simulink model "lmi_robust_maglev"  (R2018a)
settings: Solver=VariableStepAuto  StartTime=0.0  StopTime=5  RelTol=1e-3
settings Model: Creator=saad  LastModifiedBy=saad

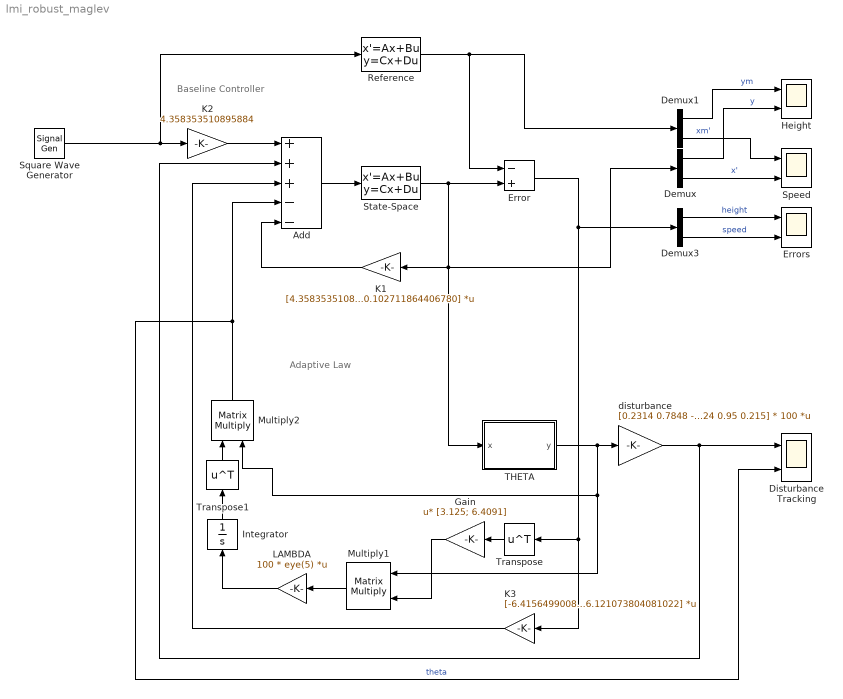
== system lmi_robust_maglev ==
  note: Adaptive Law
  note: Baseline Controller
  Add : Sum  Inputs=+++--
  Demux : Demux  Outputs=2
  Demux1 : Demux  Outputs=2
  Demux3 : Demux  Outputs=2
  Disturbance Tracking : Scope  NumInputPorts=2
  Error : Sum  Inputs=-+
  Errors : Scope  NumInputPorts=2
  Gain : Gain  Gain=[3.125; 6.4091]  Multiplication=Matrix(u*K)
  Height : Scope  NumInputPorts=2
  Integrator : Integrator
  K1 : Gain  Gain=[4.358353510895883,0.102711864406780]  Multiplication=Matrix(K*u)
  K2 : Gain  Gain=4.358353510895884
  K3 : Gain  Gain=[-6.415649900832197,-6.121073804081022]  Multiplication=Matrix(K*u)
  LAMBDA : Gain  Gain=100 * eye(5)  Multiplication=Matrix(K*u)
  Multiply1 : Product  Multiplication=Matrix(*)
  Multiply2 : Product  Multiplication=Matrix(*)
  Reference : StateSpace  A=[0,1;-3600,-84.839999999999990]  B=[0;3600]  C=eye(2)  D=[0;0]  InitialCondition=0  ContinuousStateAttributes={'angle', 'angular_speed'}
  Speed : Scope  NumInputPorts=2
  Square Wave Generator : SignalGenerator  WaveForm=square  Amplitude=-1
  State-Space : StateSpace  A=[0 1;0 0]  B=[0;826]  C=eye(2)  D=[0;0]  InitialCondition=0  ContinuousStateAttributes={'angle', 'angular_speed'}
  THETA : MATLAB Function  TreatAsAtomicUnit=on
  Transpose : Math  Operator=transpose  SaturateOnIntegerOverflow=on
  Transpose1 : Math  Operator=transpose  SaturateOnIntegerOverflow=on
  disturbance : Gain  Gain=[0.2314 0.7848 -0.624 0.95 0.215] * 100  Multiplication=Matrix(K*u)
  wires:
  Add/1 -> State-Space/1
  Square Wave Generator/1 -> Reference/1, K2/1
  K2/1 -> Add/1
  Demux/1 -> Height/2  "y"
  State-Space/1 -> Error/2, Demux/1, THETA/1(x), K1/1
  Demux1/1 -> Height/1  "ym"
  Demux1/2 -> Speed/1  "xm'"
  Reference/1 -> Error/1, Demux1/1
  THETA/1(y) -> disturbance/1, Multiply2/2, Multiply1/1
  disturbance/1 -> Add/2, Disturbance Tracking/1
  Transpose/1 -> Gain/1
  Gain/1 -> Multiply1/2
  Multiply1/1 -> LAMBDA/1
  LAMBDA/1 -> Integrator/1
  Integrator/1 -> Transpose1/1
  Transpose1/1 -> Multiply2/1
  K1/1 -> Add/5
  Multiply2/1 -> Disturbance Tracking/2, Add/4  "theta"
  K3/1 -> Add/3
  Demux3/2 -> Errors/2  "speed"
  Demux3/1 -> Errors/1  "height"
  Error/1 -> Demux3/1, K3/1, Transpose/1
  Demux/2 -> Speed/2  "x'"

== matlab function lmi_robust_maglev/THETA ==
  data: x input; y output
function y = fcn(x)

    %y = [u(1); u(2); abs(u(1))*u(2); abs(u(2))*u(2); u(1)^3];
    y = [x(1)^2; x(2); sin(x(1)) + cos(x(2)); sin(x(2)); x(1)^3];
